simulink model "multilevel"  (R2015a)
settings: Solver=ode45  StartTime=0.0  StopTime=0.02  RelTol=1e-3
libraries: powerlib x45
settings Model: TunableVars=LB,M_ma,UB,f,fit,fs,j,k,step,temp,temp1,tetha,tetha11,tetha12,tetha13,tetha14,tout,v1,v11,v1_ma,v7  TunableVarsStorageClass=Auto,Auto,Auto,Auto,Auto,Auto,Auto,Auto,Auto,Auto,Auto,Auto,Auto,Auto,Auto,Auto,Auto,Auto,Auto,Auto,Auto  TunableVarsTypeQualifier=,,,,,,,,,,,,,,,,,,,,  Creator=yahya  LastModifiedBy=yahya
settings OptimizationCC: InlineParams=on
settings RTWCC: RetainRTWFile=on

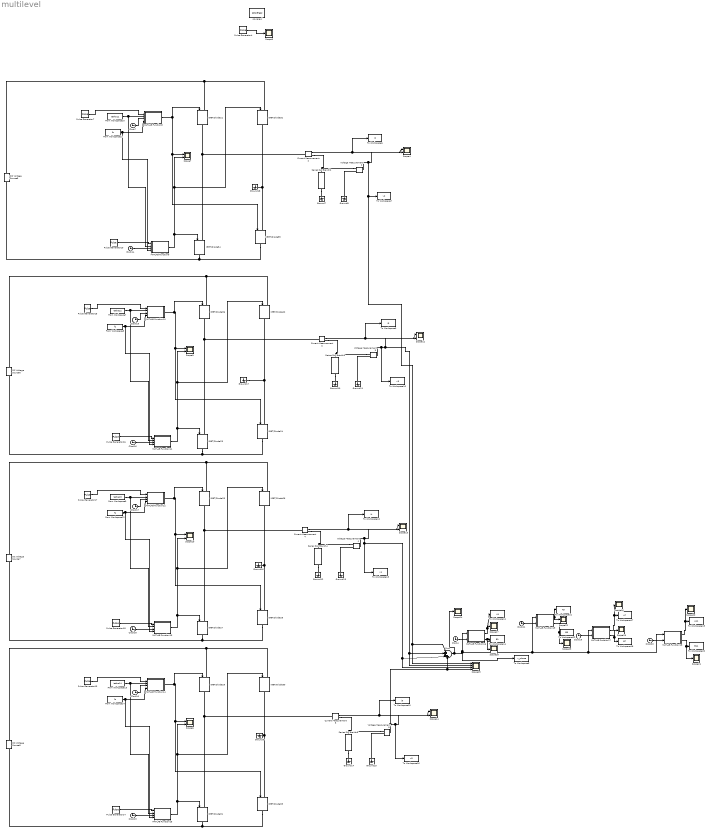
== system multilevel ==
  Clock{4,7,10,13..21} (12 alike) : Clock
  Current Measurement{2..5} (4 alike) : powerlib/Measurements/Current Measurement  PhasorSimulation=off  OutputType=Complex  PSBequivalent=0
  DC Voltage Source{5..8} (4 alike) : powerlib/Electrical Sources/DC Voltage Source  Amplitude=100  Measurements=None
  From Workspace10 : FromWorkspace  VariableName=tetha11  SampleTime=0
  From Workspace{8,11..12,14} (4 alike) : FromWorkspace  VariableName=fs  SampleTime=0
  From Workspace13 : FromWorkspace  VariableName=tetha14  SampleTime=0
  From Workspace7 : FromWorkspace  VariableName=tetha12  SampleTime=0
  From Workspace9 : FromWorkspace  VariableName=tetha13  SampleTime=0
  Ground{7..18} (12 alike) : powerlib/Elements/Ground  LConnTagsString=a
  IGBT/Diode{21..36} (16 alike) : powerlib/Power Electronics/IGBT//Diode  Ron=1e-3  Rs=1e5  Cs=inf  Measurements=off
  MATLAB Function10 : MATLAB Function  TreatAsAtomicUnit=on
  MATLAB Function11 : MATLAB Function  TreatAsAtomicUnit=on
  MATLAB Function12 : MATLAB Function  TreatAsAtomicUnit=on
  MATLAB Function13 : MATLAB Function  TreatAsAtomicUnit=on
  MATLAB Function14 : MATLAB Function  TreatAsAtomicUnit=on
  MATLAB Function15 : MATLAB Function  TreatAsAtomicUnit=on
  MATLAB Function16 : MATLAB Function  TreatAsAtomicUnit=on
  MATLAB Function17 : MATLAB Function  TreatAsAtomicUnit=on
  MATLAB Function18 : MATLAB Function  TreatAsAtomicUnit=on
  MATLAB Function19 : MATLAB Function  TreatAsAtomicUnit=on
  MATLAB Function8 : MATLAB Function  TreatAsAtomicUnit=on
  MATLAB Function9 : MATLAB Function  TreatAsAtomicUnit=on
  Pulse Generator{10,14,16,18} (4 alike) : DiscretePulseGenerator  PulseType=Time based  Amplitude=10  Period=0.02  PulseWidth=50  PhaseDelay=0.01
  Pulse Generator{7,13,15,17} (4 alike) : DiscretePulseGenerator  PulseType=Time based  Amplitude=10  Period=0.02  PulseWidth=50
  Pulse Generator4 : DiscretePulseGenerator  PulseType=Time based  Period=0.0001  PulseWidth=50
  Scope{4,6..7,9..10,12..14} (8 alike) : Scope  NumInputPorts=2
      Scope10 settings: TimeRange=1  YMin=-400~-400  YMax=400~400  SaveName=ScopeData4
      Scope12 settings: TimeRange=1  YMin=-400~-400  YMax=400~400  SaveName=ScopeData12
      Scope13 settings: TimeRange=1  YMin=-400~-400  YMax=400~400  SaveName=ScopeData13
      Scope14 settings: TimeRange=1  YMin=-400~-400  YMax=400~400  SaveName=ScopeData14
      Scope4 settings: TimeRange=1  YMin=-400~-400  YMax=400~400  SaveName=ScopeData6
      Scope6 settings: TimeRange=1  YMin=-400~-400  YMax=400~400  SaveName=ScopeData7
      Scope7 settings: TimeRange=1  YMin=-400~-400  YMax=400~400  SaveName=ScopeData9
      Scope9 settings: TimeRange=1  YMin=-400~-400  YMax=400~400  SaveName=ScopeData10
  Scope15 : Scope  NumInputPorts=4
      settings: TimeRange=1  YMin=-400~-400~-5~-5  YMax=400~400~5~5  SaveName=ScopeData15
  Scope{3,16..24} (10 alike) : Scope
      Scope16 settings: TimeRange=0.2  YMin=190  YMax=400  SaveName=ScopeData16
      Scope17 settings: TimeRange=0.2  YMin=190  YMax=400  SaveName=ScopeData17
      Scope18 settings: TimeRange=0.2  YMin=190  YMax=400  SaveName=ScopeData18
      Scope19 settings: TimeRange=0.2  YMin=190  YMax=400  SaveName=ScopeData19
      Scope20 settings: TimeRange=0.2  YMin=190  YMax=400  SaveName=ScopeData20
      Scope21 settings: TimeRange=0.2  YMin=190  YMax=400  SaveName=ScopeData21
      Scope22 settings: TimeRange=0.2  YMin=190  YMax=400  SaveName=ScopeData22
      Scope23 settings: TimeRange=0.2  YMin=190  YMax=400  SaveName=ScopeData23
      Scope24 settings: TimeRange=0.2  YMin=190  YMax=400  SaveName=ScopeData24
      Scope3 settings: TimeRange=0.03572500664993174  YMin=-1  YMax=1  SaveName=ScopeData2
  Series RLC Branch{2..5} (4 alike) : powerlib/Elements/Series RLC Branch  LConnTagsString=__new0  RConnTagsString=__new0  BranchType=R  Resistance=1  Inductance=1e-5  SetiL0=off  InitialCurrent=0  Capacitance=1e-6  Setx0=off  InitialVoltage=0  Measurements=None
  Sum : Sum  Inputs=|++++
  To Workspace10 : ToWorkspace  VariableName=v3  SaveFormat=Timeseries  SampleTime=-1
  To Workspace11 : ToWorkspace  VariableName=A1  SaveFormat=Timeseries  SampleTime=-1
  To Workspace12 : ToWorkspace  VariableName=i4  SaveFormat=Timeseries  SampleTime=-1
  To Workspace13 : ToWorkspace  VariableName=v4  SaveFormat=Timeseries  SampleTime=-1
  To Workspace14 : ToWorkspace  VariableName=B1  SaveFormat=Timeseries  SampleTime=-1
  To Workspace15 : ToWorkspace  VariableName=i5  SaveFormat=Timeseries  SampleTime=-1
  To Workspace16 : ToWorkspace  VariableName=v5  SaveFormat=Timeseries  SampleTime=-1
  To Workspace17 : ToWorkspace  VariableName=A7  SaveFormat=Timeseries  SampleTime=-1
  To Workspace18 : ToWorkspace  VariableName=B7  SaveFormat=Timeseries  SampleTime=-1
  To Workspace19 : ToWorkspace  VariableName=A11  SaveFormat=Timeseries  SampleTime=-1
  To Workspace20 : ToWorkspace  VariableName=B11  SaveFormat=Timeseries  SampleTime=-1
  To Workspace21 : ToWorkspace  VariableName=A5  SaveFormat=Timeseries  SampleTime=-1
  To Workspace22 : ToWorkspace  VariableName=B5  SaveFormat=Timeseries  SampleTime=-1
  To Workspace6 : ToWorkspace  VariableName=i2  SaveFormat=Timeseries  SampleTime=-1
  To Workspace7 : ToWorkspace  VariableName=v2  SaveFormat=Timeseries  SampleTime=-1
  To Workspace8 : ToWorkspace  VariableName=v_phase  SaveFormat=Timeseries  SampleTime=-1
  To Workspace9 : ToWorkspace  VariableName=i3  SaveFormat=Timeseries  SampleTime=-1
  Voltage Measurement{2..5} (4 alike) : powerlib/Measurements/Voltage Measurement  PhasorSimulation=off  OutputType=Complex  PSBequivalent=0
  powergui : powerlib/powergui  Priority=1  SimulationMode=Continuous  SolverType=Tustin/Backward Euler (TBE)  SampleTime=50e-6  frequency=60  SPID=off  DisableSnubberDevices=off  DisableRonSwitches=off  DisableVfSwitches=off  SwTol=0  DisplayEquations=off  Interpol=off  methode=off  Ts=100  FunctionMessages=off  echomessages=off  HookPort=off  EnableUseOfTLC=off  x0status=blocks  frequencyindice=0  Pbase=100e6  ErrMax=1e-4  Iterations=50  UnitsV=kV  UnitsW=MW  buscounter=0  RestoreLinks=warning  ResistiveCurrentMeasurement=off  Frange=[0:2:500]  Ylog=off  Xlog=on  ShowGrid=off  save=off  variable=ZData  structure=0  ZoomFFT=off  StartTime=0.0  cycles=1  DisplayStyle=1  fundamental=60  FreqAxis=off  MaxFrequency=1000  frequencyindicesteady=1  RmsSteady=1  display=off
  wires:
  Current Measurement2/1 -> To Workspace6/1, Scope4/1
  Voltage Measurement2/1 -> Sum/1, Scope15/1, To Workspace7/1, Scope4/2
  From Workspace10/1 -> MATLAB Function9/2(t), MATLAB Function8/2(t)
  From Workspace11/1 -> MATLAB Function9/4(fs), MATLAB Function8/4(fs)
  Clock7/1 -> MATLAB Function8/3(time)
  Pulse Generator7/1 -> MATLAB Function8/1(u)
  Clock14/1 -> MATLAB Function9/3(time)
  Pulse Generator10/1 -> MATLAB Function9/1(u)
  MATLAB Function8/1(y) -> IGBT/Diode21/1, IGBT/Diode35/1, Scope7/1
  MATLAB Function9/1(y) -> IGBT/Diode34/1, IGBT/Diode32/1, Scope7/2
  From Workspace7/1 -> MATLAB Function11/2(t), MATLAB Function10/2(t)
  From Workspace8/1 -> MATLAB Function11/4(fs), MATLAB Function10/4(fs)
  Clock15/1 -> MATLAB Function10/3(time)
  Pulse Generator15/1 -> MATLAB Function10/1(u)
  Clock16/1 -> MATLAB Function11/3(time)
  Pulse Generator16/1 -> MATLAB Function11/1(u)
  MATLAB Function10/1(y) -> IGBT/Diode36/1, IGBT/Diode24/1, Scope9/1
  MATLAB Function11/1(y) -> IGBT/Diode23/1, IGBT/Diode22/1, Scope9/2
  From Workspace9/1 -> MATLAB Function13/2(t), MATLAB Function12/2(t)
  From Workspace12/1 -> MATLAB Function13/4(fs), MATLAB Function12/4(fs)
  Clock17/1 -> MATLAB Function12/3(time)
  Pulse Generator17/1 -> MATLAB Function12/1(u)
  Clock18/1 -> MATLAB Function13/3(time)
  Pulse Generator18/1 -> MATLAB Function13/1(u)
  MATLAB Function12/1(y) -> IGBT/Diode25/1, IGBT/Diode28/1, Scope10/1
  MATLAB Function13/1(y) -> IGBT/Diode27/1, IGBT/Diode26/1, Scope10/2
  From Workspace13/1 -> MATLAB Function15/2(t), MATLAB Function14/2(t)
  From Workspace14/1 -> MATLAB Function15/4(fs), MATLAB Function14/4(fs)
  Clock10/1 -> MATLAB Function14/3(time)
  Pulse Generator13/1 -> MATLAB Function14/1(u)
  Clock13/1 -> MATLAB Function15/3(time)
  Pulse Generator14/1 -> MATLAB Function15/1(u)
  MATLAB Function14/1(y) -> IGBT/Diode29/1, IGBT/Diode33/1, Scope6/1
  MATLAB Function15/1(y) -> IGBT/Diode31/1, IGBT/Diode30/1, Scope6/2
  Current Measurement3/1 -> To Workspace9/1, Scope12/1
  Voltage Measurement3/1 -> Sum/2, Scope15/2, Scope12/2, To Workspace10/1
  Current Measurement4/1 -> To Workspace12/1, Scope13/1
  Voltage Measurement4/1 -> Scope15/3, Sum/3, To Workspace13/1, Scope13/2
  Current Measurement5/1 -> To Workspace15/1, Scope14/1
  Voltage Measurement5/1 -> Sum/4, Scope15/4, To Workspace16/1, Scope14/2
  Clock4/1 -> MATLAB Function16/2(time)
  MATLAB Function16/1(A1) -> To Workspace11/1, Scope17/1
  MATLAB Function16/2(B1) -> Scope18/1, To Workspace14/1
  Clock19/1 -> MATLAB Function17/2(time)
  MATLAB Function17/1(A7) -> Scope16/1, To Workspace17/1
  MATLAB Function17/2(B7) -> To Workspace18/1, Scope19/1
  Sum/1 -> Scope24/1, MATLAB Function18/1(u), MATLAB Function17/1(u), MATLAB Function19/1(u), To Workspace8/1, MATLAB Function16/1(u)
  Clock20/1 -> MATLAB Function18/2(time)
  MATLAB Function18/1(A11) -> Scope20/1, To Workspace19/1
  MATLAB Function18/2(B11) -> Scope21/1, To Workspace20/1
  Clock21/1 -> MATLAB Function19/2(time)
  MATLAB Function19/1(A5) -> Scope22/1, To Workspace21/1
  MATLAB Function19/2(B5) -> Scope23/1, To Workspace22/1
  Pulse Generator4/1 -> Scope3/1
  connections:
  IGBT/Diode21/LConn1 -- DC Voltage Source5/RConn1 -- IGBT/Diode32/LConn1
  DC Voltage Source5/LConn1 -- IGBT/Diode34/RConn1 -- IGBT/Diode35/RConn1
  Voltage Measurement2/LConn1 -- Series RLC Branch2/LConn1 -- Current Measurement2/RConn1
  Current Measurement2/LConn1 -- IGBT/Diode21/RConn1 -- IGBT/Diode34/LConn1
  IGBT/Diode36/LConn1 -- DC Voltage Source6/RConn1 -- IGBT/Diode22/LConn1
  DC Voltage Source6/LConn1 -- IGBT/Diode23/RConn1 -- IGBT/Diode24/RConn1
  IGBT/Diode36/RConn1 -- IGBT/Diode23/LConn1 -- Current Measurement3/LConn1
  IGBT/Diode25/LConn1 -- DC Voltage Source7/RConn1 -- IGBT/Diode26/LConn1
  DC Voltage Source7/LConn1 -- IGBT/Diode27/RConn1 -- IGBT/Diode28/RConn1
  IGBT/Diode22/RConn1 -- IGBT/Diode24/LConn1 -- Ground17/LConn1
  IGBT/Diode29/LConn1 -- DC Voltage Source8/RConn1 -- IGBT/Diode30/LConn1
  IGBT/Diode31/RConn1 -- DC Voltage Source8/LConn1 -- IGBT/Diode33/RConn1
  IGBT/Diode26/RConn1 -- IGBT/Diode28/LConn1 -- Ground16/LConn1
  IGBT/Diode30/RConn1 -- IGBT/Diode33/LConn1 -- Ground9/LConn1
  IGBT/Diode32/RConn1 -- IGBT/Diode35/LConn1 -- Ground18/LConn1
  Current Measurement4/LConn1 -- IGBT/Diode27/LConn1 -- IGBT/Diode25/RConn1
  IGBT/Diode29/RConn1 -- IGBT/Diode31/LConn1 -- Current Measurement5/LConn1
  Voltage Measurement3/LConn1 -- Series RLC Branch3/LConn1 -- Current Measurement3/RConn1
  Voltage Measurement4/LConn1 -- Series RLC Branch4/LConn1 -- Current Measurement4/RConn1
  Voltage Measurement5/LConn1 -- Series RLC Branch5/LConn1 -- Current Measurement5/RConn1
  Series RLC Branch4/RConn1 -- Ground12/LConn1
  Series RLC Branch5/RConn1 -- Ground14/LConn1
  Series RLC Branch3/RConn1 -- Ground10/LConn1
  Voltage Measurement4/LConn2 -- Ground13/LConn1
  Series RLC Branch2/RConn1 -- Ground7/LConn1
  Voltage Measurement5/LConn2 -- Ground15/LConn1
  Voltage Measurement2/LConn2 -- Ground8/LConn1
  Voltage Measurement3/LConn2 -- Ground11/LConn1

== matlab function multilevel/MATLAB Function10 ==
  data: u input; y output; t input; time input; fs input
function y = fcn(u,t,time,fs)
%#codegen
Q = fs;
z1 = mod(time,fs);
t1 = time-z1;
w = (t1/fs)+1;
fs = (fs*w)-(fs/2);
z = (fs)-t;
fs = fs-(Q/2);
t = t+fs;
if u > 0 && t <= time && time <= z
    y = u;
else
    y = 0;
end
end

== matlab function multilevel/MATLAB Function11 ==
  data: u input; y output; t input; time input; fs input
function y = fcn(u,t,time,fs)
%#codegen
Q = fs/2;
z1 = mod(time,fs);
t1 = time-z1;
w = (t1/fs)+1;
fs = (fs*w);
z = (fs)-t;
t = t+fs-Q;
if t <= time && time <= z
    y = u;
else
    y = 0;
end
end

== matlab function multilevel/MATLAB Function12 ==
  data: u input; y output; t input; time input; fs input
function y = fcn(u,t,time,fs)
%#codegen
Q = fs;
z1 = mod(time,fs);
t1 = time-z1;
w = (t1/fs)+1;
fs = (fs*w)-(fs/2);
z = (fs)-t;
fs = fs-(Q/2);
t = t+fs;
if u > 0 && t <= time && time <= z
    y = u;
else
    y = 0;
end
end

== matlab function multilevel/MATLAB Function13 ==
  data: u input; y output; t input; time input; fs input
function y = fcn(u,t,time,fs)
%#codegen
Q = fs/2;
z1 = mod(time,fs);
t1 = time-z1;
w = (t1/fs)+1;
fs = (fs*w);
z = (fs)-t;
t = t+fs-Q;
if t <= time && time <= z
    y = u;
else
    y = 0;
end
end

== matlab function multilevel/MATLAB Function14 ==
  data: u input; y output; t input; time input; fs input
function y = fcn(u,t,time,fs)
%#codegen
Q = fs;
z1 = mod(time,fs);
t1 = time-z1;
w = (t1/fs)+1;
fs = (fs*w)-(fs/2);
z = (fs)-t;
fs = fs-(Q/2);
t = t+fs;
if u > 0 && t <= time && time <= z
    y = u;
else
    y = 0;
end
end

== matlab function multilevel/MATLAB Function15 ==
  data: u input; y output; t input; time input; fs input
function y = fcn(u,t,time,fs)
%#codegen
Q = fs/2;
z1 = mod(time,fs);
t1 = time-z1;
w = (t1/fs)+1;
fs = (fs*w);
z = (fs)-t;
t = t+fs-Q;
if t <= time && time <= z
    y = u;
else
    y = 0;
end
end

== matlab function multilevel/MATLAB Function8 ==
  data: u input; y output; t input; time input; fs input
function y = fcn(u,t,time,fs)
%#codegen
Q = fs;
z1 = mod(time,fs);
t1 = time-z1;
w = (t1/fs)+1;
fs = (fs*w)-(fs/2);
z = (fs)-t;
fs = fs-(Q/2);
t = t+fs;
if u > 0 && t <= time && time <= z
    y = u;
else
    y = 0;
end
end

== matlab function multilevel/MATLAB Function9 ==
  data: u input; y output; t input; time input; fs input
function y = fcn(u,t,time,fs)
%#codegen
Q = fs/2;
z1 = mod(time,fs);
t1 = time-z1;
w = (t1/fs)+1;
fs = (fs*w);
z = (fs)-t;
t = t+fs-Q;
if t <= time && time <= z
    y = u;
else
    y = 0;
end
end

== matlab function multilevel/MATLAB Function16 ==
  data: u input; A1 output; time input; B1 output
function [A1,B1] = fcn(u,time)
%#codegen
A1 = u*sin(2*pi*50*time);
B1 = u*cos(2*pi*50*time);
end

== matlab function multilevel/MATLAB Function17 ==
  data: u input; A7 output; time input; B7 output
function [A7,B7] = fcn(u,time)
%#codegen
A7 = u*sin(7*2*pi*50*time);
B7 = u*cos(7*2*pi*50*time);
end

== matlab function multilevel/MATLAB Function18 ==
  data: u input; A11 output; time input; B11 output
function [A11,B11] = fcn(u,time)
%#codegen
A11 = u*sin(11*2*pi*50*time);
B11 = u*cos(11*2*pi*50*time);
end

== matlab function multilevel/MATLAB Function19 ==
  data: u input; A5 output; time input; B5 output
function [A5,B5] = fcn(u,time)
%#codegen
A5 = u*sin(5*2*pi*50*time);
B5 = u*cos(5*2*pi*50*time);
end
